simulink model "Observer_State_Feedback_nonlinear_1"  (R2016b)
settings: Solver=FixedStepAuto  StartTime=0.0  StopTime=5  FixedStep=.01  RelTol=1e-3
settings Model: Creator=imi  LastModifiedBy=imi

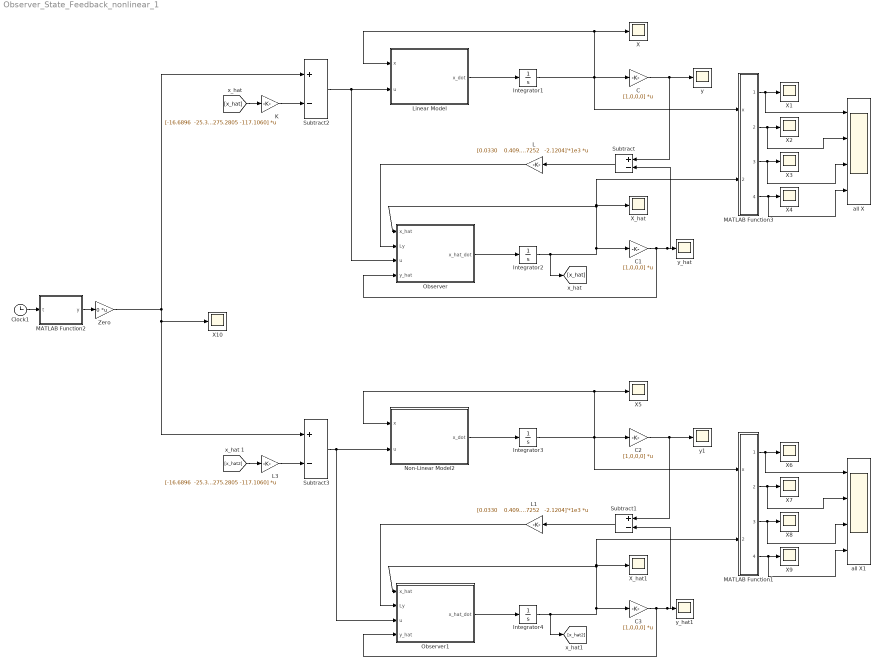
== system Observer_State_Feedback_nonlinear_1 ==
  C{,1..3} (4 alike) : Gain  Gain=[1,0,0,0]  Multiplication=Matrix(K*u)
  Clock1 : Clock
  Integrator1 : Integrator  InitialCondition=zeros(4,1)
  Integrator2 : Integrator  InitialCondition=[.1;.2;.3;.4]*0.1
  Integrator3 : Integrator  InitialCondition=zeros(4,1)
  Integrator4 : Integrator  InitialCondition=[.1;.2;.3;.4]*.01
  K : Gain  Gain="[-16.6896  -25.3522 -275.2805 -117.1060]"  Multiplication=Matrix(K*u)
  L : Gain  Gain="[0.0330    0.4093   -0.7252   -2.1204]'*1e3"  Multiplication=Matrix(K*u)
  L1 : Gain  Gain="[0.0330    0.4093   -0.7252   -2.1204]'*1e3"  Multiplication=Matrix(K*u)
  L3 : Gain  Gain="[-16.6896  -25.3522 -275.2805 -117.1060]"  Multiplication=Matrix(K*u)
  Linear Model : MATLAB Function  TreatAsAtomicUnit=on
  MATLAB Function1 : MATLAB Function  TreatAsAtomicUnit=on
  MATLAB Function2 : MATLAB Function  TreatAsAtomicUnit=on
  MATLAB Function3 : MATLAB Function  TreatAsAtomicUnit=on
  Non-Linear Model2 : MATLAB Function  TreatAsAtomicUnit=on
  Observer : MATLAB Function  TreatAsAtomicUnit=on
  Observer1 : MATLAB Function  TreatAsAtomicUnit=on
  Subtract{,1..3} (4 alike) : Sum  Inputs=+-
  X{,1..10} (11 alike) : Scope
  X_hat : Scope
  X_hat1 : Scope
  Zero : Gain  Gain=0  Multiplication=Matrix(K*u)
  all X : Scope  NumInputPorts=4
  all X1 : Scope  NumInputPorts=4
  y : Scope
  y1 : Scope
  y_hat : Scope
  y_hat1 : Scope
  wires:
  Linear Model/1(x_dot) -> Integrator1/1
  Integrator2/1 -> [x_hat], C1/1, MATLAB Function3/2(x_hat), X_hat/1, Observer/1(x_hat)
  Observer/1(x_hat_dot) -> Integrator2/1
  L/1 -> Observer/2(Ly)
  C/1 -> y/1, Subtract/1
  C1/1 -> Subtract/2, y_hat/1, Observer/4(y_hat)
  MATLAB Function3/1(x1) -> all X/1, X1/1
  MATLAB Function3/2(x2) -> all X/2, X2/1
  MATLAB Function3/3(x3) -> all X/3, X3/1
  Integrator1/1 -> Linear Model/1(x), X/1, MATLAB Function3/1(x), C/1
  MATLAB Function3/4(x4) -> all X/4, X4/1
  Subtract/1 -> L/1
  Clock1/1 -> MATLAB Function2/1(t)
  Subtract2/1 -> Observer/3(u), Linear Model/2(u)
  [x_hat] -> K/1
  MATLAB Function2/1(y) -> Zero/1
  K/1 -> Subtract2/2
  Non-Linear Model2/1(x_dot) -> Integrator3/1
  Integrator4/1 -> Observer1/1(x_hat), X_hat1/1, MATLAB Function1/2(x_hat), C3/1, [x_hat2]
  Observer1/1(x_hat_dot) -> Integrator4/1
  L1/1 -> Observer1/2(Ly)
  C2/1 -> Subtract1/1, y1/1
  C3/1 -> Observer1/4(y_hat), y_hat1/1, Subtract1/2
  MATLAB Function1/1(x1) -> X6/1, all X1/1
  MATLAB Function1/2(x2) -> X7/1, all X1/2
  MATLAB Function1/3(x3) -> X8/1, all X1/3
  Integrator3/1 -> C2/1, MATLAB Function1/1(x), Non-Linear Model2/1(x), X5/1
  MATLAB Function1/4(x4) -> X9/1, all X1/4
  Subtract1/1 -> L1/1
  Subtract3/1 -> Non-Linear Model2/2(u), Observer1/3(u)
  [x_hat2] -> L3/1
  L3/1 -> Subtract3/2
  Zero/1 -> X10/1, Subtract3/1, Subtract2/1

== matlab function Observer_State_Feedback_nonlinear_1/Linear Model ==
  data: x input; u input; x_dot output
function x_dot = fcn(x,u)

m1=.5;
m2=.5;
m=.25;
g=9.8;
M=2;
A=[0,1,0,0;
    0,0,-m1*m2*g/(1-m1*m2),0;
    0,0,0,1;
    0,0,m2*g/(1-m1*m2),0];

B=[0;
    1/(m+M)/(1-m1*m2);
    0;
    -m2/(m+M);];
    
x_dot=A*x+B*u;

== matlab function Observer_State_Feedback_nonlinear_1/Observer ==
  data: x_hat input; Ly input; u input; x_hat_dot output; y_hat input
function x_hat_dot = fcn(x_hat,Ly,u,y_hat)

m1=.5;
m2=.5;
m=.25;
g=9.8;
M=2;
A=[0,1,0,0;
    0,0,-m1*m2*g/(1-m1*m2),0;
    0,0,0,1;
    0,0,m2*g/(1-m1*m2),0];



B=[0;
    1/(m+M)/(1-m1*m2);
    0;
    -m2/(m+M);];
    


x_hat_dot=A*x_hat+B*u+(Ly);

== matlab function Observer_State_Feedback_nonlinear_1/MATLAB Function3 ==
  data: x input; x_hat input; x1 output; x2 output; x3 output; x4 output
function [x1,x2,x3,x4] = CP(x,x_hat)

x1=[x(1),x_hat(1)];
x2=[x(2),x_hat(2)];
x3=[x(3),x_hat(3)];
x4=[x(4),x_hat(4)];

== matlab function Observer_State_Feedback_nonlinear_1/MATLAB Function1 ==
  data: x input; x_hat input; x1 output; x2 output; x3 output; x4 output
function [x1,x2,x3,x4] = CP(x,x_hat)

x1=[x(1),x_hat(1)];
x2=[x(2),x_hat(2)];
x3=[x(3),x_hat(3)];
x4=[x(4),x_hat(4)];

== matlab function Observer_State_Feedback_nonlinear_1/Observer1 ==
  data: x_hat input; Ly input; u input; x_hat_dot output; y_hat input
function x_hat_dot = fcn(x_hat,Ly,u,y_hat)

m1=.5;
m2=.5;
m=.25;
g=9.8;
M=2;
A=[0,1,0,0;
    0,0,-m1*m2*g/(1-m1*m2),0;
    0,0,0,1;
    0,0,m2*g/(1-m1*m2),0];



B=[0;
    1/(m+M)/(1-m1*m2);
    0;
    -m2/(m+M);];
    


x_hat_dot=A*x_hat+B*u+(Ly);

== matlab function Observer_State_Feedback_nonlinear_1/MATLAB Function2 ==
  data: t input; y output
function y = fcn(t)
if(t<6)
    y=.1;
else
    y=.15;
end

== matlab function Observer_State_Feedback_nonlinear_1/Non-Linear Model2 ==
  data: x input; u input; x_dot output
function x_dot = fcn(x,u)


m1=.5;
m2=.5;
m=.25;
g=9.8;
M=2;

x_1_d=x(2);
x_2_d=-m1*m2*g*cos(x(3))*sin(x(3))/[1-m1*m2*(cos(x(3)))^2]...
    +m1*sin(x(3))*(x(4))^2/[1-m1*m2*(cos(x(3)))^2]...
    +1/(m+M)/[1-m1*m2*(cos(x(3)))^2]*u;
x_3_d=x(4);
x_4_d=g*m2*sin(x(3))/[1-m1*m2*(cos(x(3)))^2]...
    -m1*m2*(cos(x(3))*sin(x(3)))*(x(4))^2/[1-m1*m2*(cos(x(3)))^2]...
    -m2*cos(x(3))/(m+M)/[1-m1*m2*(cos(x(3)))^2]*u;

    
x_dot=[x_1_d;x_2_d;x_3_d;x_4_d];
